simulink library "Collector_EN12975_CONF"  (R2016b)
settings: Solver=ode45  StartTime=0.0  StopTime=10.0  RelTol=1e-3  EnableMultiTasking=on
undefined symbols (not defined in the file): Acol, Ncollector, path_carnot, Qdot, THBin, THBout
libraries: carnot x2
settings Model: Creator=lena.frank  LastModifiedBy=drhf
settings DataIOCC: LimitDataPoints=on  SaveFormat=Array  SignalLoggingSaveFormat=ModelDataLogs
settings OptimizationCC: ExpressionDepthLimit=2147483647  LifeSpan=inf
settings DebuggingCC: UnderspecifiedInitializationDetection=Classic  MergeDetectMultiDrivingBlocksExec=none  SolverPrmCheckMsg=warning  FcnCallInpInsideContextMsg=warning  StateNameClashWarn=warning  SFUnexpectedBacktrackingDiag=warning  SFNoUnconditionalDefaultTransitionDiag=warning  SFExecutionAtInitializationDiag=none
settings HardwareCC: ProdBitPerPointer=32  ProdBitPerSizeT=32  ProdBitPerPtrDiffT=32  ProdLargestAtomicFloat=None  ProdIntDivRoundTo=Undefined  ProdEndianess=Unspecified  ProdWordSize=32  ProdHWDeviceType=32-bit Generic
settings ModelReferenceCC: PropagateSignalLabelsOutOfModel=off
settings GRTTargetCC: TargetLangStandard=C89/C90 (ANSI)  GeneratePreprocessorConditionals=Disable all  CombineOutputUpdateFcns=off  GRTInterface=on
settings ConfigComp: CovMetricSettings=dw  CovHtmlReporting=on  CovSaveCumulativeToWorkspaceVar=on  CovSaveSingleToWorkspaceVar=on  CovExternalEMLEnable=off

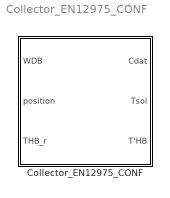
== system Collector_EN12975_CONF ==
  Collector_EN12975_CONF : Subsystem  mask(configurated Solar Thermal Collector){tini=20, Ncollector=Ncollector, PathName=fullfile(path_carnot('libsl'), 'Source','Solar_Thermal','Collector_EN12975_CONF','parameter_set'), FileName='DefaultCollector.mat', userPath=off, userParam=off, acol=3.5, len=0.1, fta=0.7, c1=0.7, c2=0.001, c3=0, c4=0, c5=7000, c6=0, KbAngles=[0 5 10 15 20 25 30 35 40 45 50 55 60 65 70 75 80 85 90], KbL=[1 1 0.9999 0.9996 0.9991 0.9982 0.9965 0.9935 0.9886 0.9807 0.9678 0.9473 0.9148 0.8638 0.7846 0.6644 0.4907 0.2599 0], KbT=[1 1 1 1 1 1 1 1 1 1 1 0.875 0.75 0.625 0.5 0.375 0.25 0.125 0], Kd=0.92, dplin=10, dpqua=10, SensorTimeConstant=10}
      mask prompts: tini "Initial temperature [°C]"; Ncollector "Number of collectors in parallel"; PathName "Path"; FileName "Parameter set"; userPath "Edit path and name of parameter set"; userParam "User defined parameters"; acol "A : collector surface  [m²]"; len "length between inlet and outlet [m]"; fta "F'(TauAlfa)"; c1 "c1 : heat loss coefficient at (Tm-Ta)=0  [W/(m²*K)]"; c2 "c2: temperature dependence of the heat loss coefficient [W/(m*K)²]"; c3 "c3 : wind speed dependence of the heat loss coefficient [J/(m³K)]"; c4 "c4 : sky temperature dependence of the heat loss coefficient [W/(m²K)]"; c5 "c5 : effective thermal capacity [J/(m²K)]"; c6 "c6 : wind dependence of conversion factor [s/m]"; KbAngles "Kb: angles for longitudinal and transversal IAM [degree]"; KbL "Kb(L) : incident angle modifier in longitudinal plane (beam radiation)"; KbT "Kb(T) : incident angle modifier in transversal plane (beam radiation)"; Kd "Kd : Incidence angle modifier diffuse radiation"; dplin "linear pressure drop in Pa/(kg/s)"; dpqua "quadratic pressure drop in Pa/(kg/s)²"; SensorTimeConstant "time constant of sensor [s]"
      mask help:
      | Dynamic 1-node collector model according to EN 12975 standard.
      | This block uses predefined parameter sets.
      mask init:
      | % callback to set parameters of model
      | [ok, param] = CarnotCallbacks_CollectorEN12975Conf('SetParameters',gcbh,PathName,FileName);
      mask Help: web(fullfile(path_carnot('help'),'collector_en12975.html'),'-helpbrowser')
      mask TypeOptions tini: Collector_EN12975/tini | T_Sensor/t0
      mask TypeOptions Ncollector: Ncollector/Value
      mask Callback userPath: [ok, param] = CarnotCallbacks_CollectorEN12975Conf('UserEdit',gcbh);
      mask Callback userParam: [ok, param] = CarnotCallbacks_CollectorEN12975Conf('UserEdit',gcbh);
      mask TypeOptions acol: Collector_EN12975/acol
      mask TypeOptions len: Collector_EN12975/len
      mask TypeOptions fta: Collector_EN12975/fta
      mask TypeOptions c1: Collector_EN12975/c1
      mask TypeOptions c2: Collector_EN12975/c2
      mask TypeOptions c3: Collector_EN12975/c3
      mask TypeOptions c4: Collector_EN12975/c4
      mask TypeOptions c5: Collector_EN12975/c5
      mask TypeOptions c6: Collector_EN12975/c6
      mask TypeOptions KbAngles: Collector_EN12975/kblangle | Collector_EN12975/kbtangle
      mask TypeOptions KbL: Collector_EN12975/KbL
      mask TypeOptions KbT: Collector_EN12975/KbT
      mask TypeOptions Kd: Collector_EN12975/Kd
      mask TypeOptions dplin: Collector_EN12975/lin
      mask TypeOptions dpqua: Collector_EN12975/qua
      mask TypeOptions SensorTimeConstant: T_Sensor/tc
      mask DialogControl ParameterGroupVar Prompt: Picking a parameter set
      mask DialogControl Control2 Prompt: Carnot public data
      mask DialogControl Control2 Callback: [ok, file] = CarnotCallbacks_CollectorEN12975Conf('GetFilename',gcbh,'public');
      mask DialogControl Control3 Prompt: Carnot internal data
      mask DialogControl Control3 Callback: [ok, file] = CarnotCallbacks_CollectorEN12975Conf('GetFilename',gcbh,'internal');
      mask DialogControl Control4 Prompt: Selected path
      mask DialogControl Control4 Callback: [ok, file] = CarnotCallbacks_CollectorEN12975Conf('GetFilename',gcbh,'selected');
      mask DialogControl Control5 Prompt: Save in Carnot interal data
      mask DialogControl Control5 Callback: [ok, param] = CarnotCallbacks_CollectorEN12975Conf('SaveFilename',gcbh,'internal','COL');
      mask DialogControl Control6 Prompt: Save in seleced path
      mask DialogControl Control6 Callback: [ok, param] = CarnotCallbacks_CollectorEN12975Conf('SaveFilename',gcbh,'selected','COL');
      mask Display:
      | % user defined picture file
      | picfile = fullfile(path_carnot('intlibsl'), ...
      |     'Source','Solar_Thermal','Collector_EN12975_CONF','parameter_set', ...
      |      'Collector_CONF.jpg');
      | 
      | pic = false;
      | 
      | % show internal picture if defined
      | if ~BlockIsInCarnotLibrary    % if not located in library any more
      |     if exist(picfile)
      |         image(imread(picfile), [0.2, 0, 0.6, 1])
      |         set_param(gcb, 'BackgroundColor', 'White')
      |         pic = true;
      |     end
      | end
      | 
      | if ~pic    % show public picture
      |     disp('solar thermal\ncollector\nEN 12975\nIAM-Table')
      |     set_param(gcb, 'BackgroundColor', 'Yellow')
      | end
      | 
      | % Show port labels: same as port labels in the subsystem,
      | % but display with a picture covers the text. Have to reprint it.
      | % port_label('input',1,'WDB')
      | % port_label('input',2,'position')
      | % port_label('input',3,'THB_r')
      | % port_label('output',1,'Cdat')
      | % port_label('output',2,'Tsol')
      | % port_label('output',3,'THB_s')

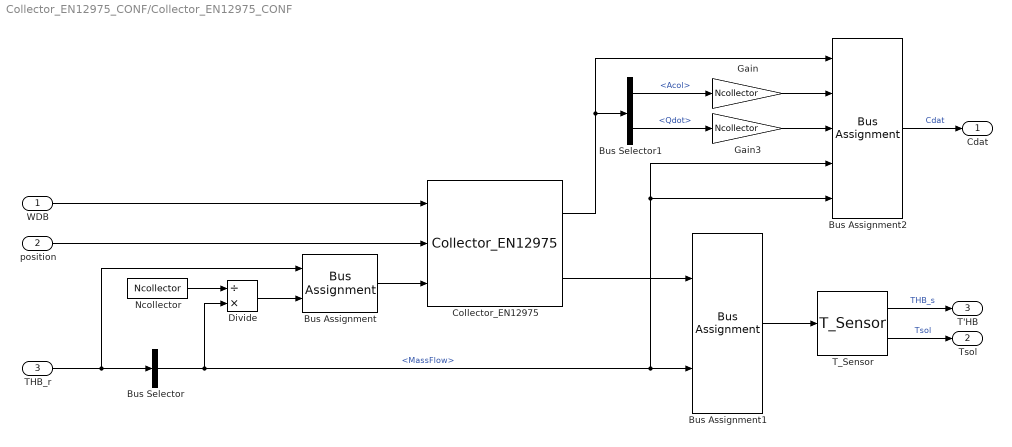
== system Collector_EN12975_CONF/Collector_EN12975_CONF ==
  WDB : Inport
  position : Inport  Port=2
  THB_r : Inport  Port=3
  Bus Assignment : BusAssignment  AssignedSignals=MassFlow
  Bus Assignment1 : BusAssignment  AssignedSignals=MassFlow
  Bus Assignment2 : BusAssignment  AssignedSignals=Acol,Qdot,THBin.MassFlow,THBout.MassFlow
  Bus Selector : BusSelector  OutputSignals=MassFlow
  Bus Selector1 : BusSelector  OutputSignals=Acol,Qdot
  Collector_EN12975 : carnot/Source/Solar_Thermal/Collector_EN12975  acol=acol  len=len  fta=fta  c1=c1  c2=c2  c3=c3  c4=c4  c5=c5  c6=c6  kblangle=KbAngles  KbL=KbL  kbtangle=KbAngles  KbT=KbT  Kd=Kd  lin=dplin  qua=dpqua  tini=tini
  Divide : Product  Inputs=/*
  Gain : Gain  Gain=Ncollector
  Gain3 : Gain  Gain=Ncollector
  Ncollector : Constant  Value=Ncollector
  T_Sensor : carnot/Control/T_Sensor  tc=SensorTimeConstant  t0=tini
  Cdat : Outport
  Tsol : Outport  Port=2
  T'HB : Outport  Port=3
  wires:
  T_Sensor/1 -> T'HB/1  "THB_s"
  T_Sensor/2 -> Tsol/1  "Tsol"
  Bus Assignment2/1 -> Cdat/1  "Cdat"
  Gain3/1 -> Bus Assignment2/3
  Gain/1 -> Bus Assignment2/2
  Bus Selector1/2 -> Gain3/1  "<Qdot>"
  Bus Selector1/1 -> Gain/1  "<Acol>"
  Divide/1 -> Bus Assignment/2
  Ncollector/1 -> Divide/1
  Bus Selector/1 -> Bus Assignment1/2, Bus Assignment2/4, Bus Assignment2/5, Divide/2  "<MassFlow>"
  Bus Assignment1/1 -> T_Sensor/1
  Bus Assignment/1 -> Collector_EN12975/3
  Collector_EN12975/1 -> Bus Selector1/1, Bus Assignment2/1
  THB_r/1 -> Bus Selector/1, Bus Assignment/1
  position/1 -> Collector_EN12975/2
  WDB/1 -> Collector_EN12975/1
  Collector_EN12975/2 -> Bus Assignment1/1
